simulink model "Practica4"  (R2024b)
settings: Solver=VariableStepAuto  StartTime=0.0  StopTime=1  MaxStep=1e-4  RelTol=1e-3
values from neighbouring files (symbols this model uses):
  C1 = 10e-3    (= 0.01)    [Practica4_Datos.m]    (also in Practica_4.m)
  C2 = 600e-6    (= 0.0006)    [Practica4_Datos.m]    (also in Practica_4.m)
  f = 20e3    (= 20000)    [ApartadoB.m]    (also in ApartadoB_Datos.m; ApartadoC.m = 8000; Practica4_Datos.m = 16000; Practica_4.m = 16000)
  L = 4e-3    (= 0.004)    [ApartadoB.m]    (also in ApartadoB_Datos.m; Practica4_Datos.m = 0.005; Practica_4.m = 0.005)
  L1 = 0    [ApartadoC.m]    (also in Practica4_Datos.m; Practica_4.m)
  L2 = 0    [ApartadoC.m]    (also in Practica4_Datos.m; Practica_4.m)
  Lm = 0    [ApartadoC.m]    (also in Practica4_Datos.m; Practica_4.m)
  Pmp = 10524.2    [ApartadoC.m]    (also in Practica4_Datos.m = 4037.5; Practica_4.m = 4037.5)
  R1 = 0.1    [ApartadoC.m]    (also in Practica4_Datos.m; Practica_4.m)
  R2 = 0.1    [ApartadoC.m]    (also in Practica4_Datos.m; Practica_4.m)
  RL = VdcLinkDes.^2/Pnom    [Practica4_Datos.m]    (also in Practica_4.m)
  Rm = 10e6    (= 10000000)    [ApartadoC.m]    (also in Practica4_Datos.m; Practica_4.m)
  T = 1/f    (= 5e-05)    [ApartadoB.m]    (also in ApartadoB_Datos.m; ApartadoC.m = 0.000125; Practica4_Datos.m = 6.25e-05; Practica_4.m = 6.25e-05)
  V1 = V2/2    (= 200)    [ApartadoC.m]    (also in Practica4_Datos.m; Practica_4.m)
  V2 = 400    [ApartadoC.m]    (also in Practica4_Datos.m; Practica_4.m)
  VdcLinkDes = 800    [Practica4_Datos.m]    (also in Practica_4.m)
  Vmp = 223.836    [ApartadoC.m]    (also in Practica4_Datos.m = 207; Practica_4.m = 207)
libraries: spsParallelRLCBranchLib x9, spsDiodeLib x8, spsCurrentMeasurementLib x6, spsVoltageMeasurementLib x3, slpidlib x2, spsIGBTLib x2, simulink x2, spsLinearTransformerLib x1, spsBistableLib x1, spsPVArrayLib x1, spsThreePhaseProgrammableVoltageSourceLib x1, sps_lib x1
settings Model: Creator=javier  LastModifiedBy=javier

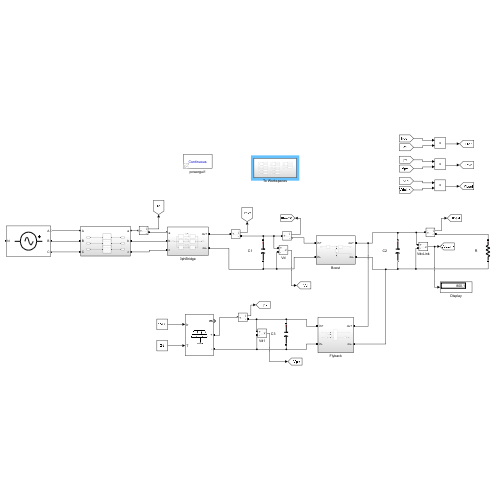
[thumbnail: Simulink's stored preview of the top-level diagram]
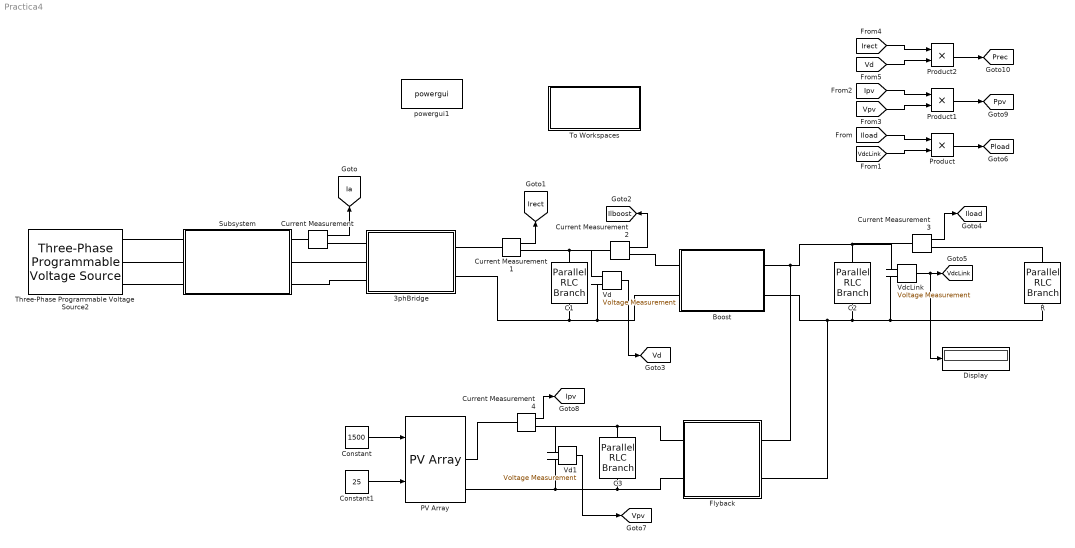
== system Practica4 ==
  3phBridge : Subsystem
  Boost : Subsystem
  C1 : spsParallelRLCBranchLib/Parallel RLC Branch  LConnTagsString=a  RConnTagsString=__new0  BranchType=C  Resistance=30  Inductance=1e-3  SetiL0=off  InitialCurrent=0  Capacitance=C1  Setx0=on  InitialVoltage=VoC1  Measurements=None
  C2 : spsParallelRLCBranchLib/Parallel RLC Branch  LConnTagsString=a  RConnTagsString=__new0  BranchType=C  Resistance=30  Inductance=1e-3  SetiL0=off  InitialCurrent=0  Capacitance=C2  Setx0=on  InitialVoltage=VoC2  Measurements=None
  C3 : spsParallelRLCBranchLib/Parallel RLC Branch  LConnTagsString=a  RConnTagsString=__new0  BranchType=C  Resistance=30  Inductance=1e-3  SetiL0=off  InitialCurrent=0  Capacitance=1.5e-3  Setx0=off  InitialVoltage=0  Measurements=None
  Constant : Constant  Value=1500
  Constant1 : Constant  Value=25
  Current Measurement{,1..4} (5 alike) : spsCurrentMeasurementLib/Current Measurement  PhasorSimulation=off  OutputType=Complex  PSBequivalent=0
  Display : Display
  Flyback : Subsystem
  PV Array : spsPVArrayLib/PV Array  Npar=3  Nser=6  PlotType=array @ 25 deg.C & specified irradiances  S_vec=[1500]  Temp_C_vec=[25]  ModuleName=Advance Solar Hydro Wind Power API-150  PlotWhenSelected=off  Pm=150.075  Ncell=72  Voc=41.8  Isc=5.05  Vm=34.5  Im=4.35  beta_Voc_pc=-0.419  alpha_Isc_pc=0.096  beta_Voc=-0.17514  alpha_Isc=0.004848  IL=5.0762  I0=1.155e-09  nI=1.0233  Rsh=71.9537  Rs=0.37337  RobustModel=off  RobustCellTemperature=313.3991  BAL=on  Tc=1e-6  Tfilter=5e-5
  Product : Product
  Product1 : Product
  Product2 : Product
  R : spsParallelRLCBranchLib/Parallel RLC Branch  LConnTagsString=a  RConnTagsString=__new0  BranchType=R  Resistance=RL  Inductance=1e-3  SetiL0=off  InitialCurrent=0  Capacitance=10e-3  Setx0=off  InitialVoltage=0  Measurements=None
  Subsystem : Subsystem
  Three-Phase Programmable Voltage Source2 : spsThreePhaseProgrammableVoltageSourceLib/Three-Phase Programmable Voltage Source  PositiveSequence="[400  0 50]"  VariationEntity=None  VariationType=Table of time-amplitude pairs  VariationTypeAlt=Step  VariationStep=0.5  VariationRate=10  VariationMagnitude=0.3  VariationFrequency=2  VariationTiming=[1 2]  VariationPhaseA=off  Amplitudes=[1 0.8 1.2 1.0]  TimeValues=[0 0.1 0.15 0.2]  HarmonicGeneration=off  HarmonicA=[3 0.2 -25 0]  HarmonicB=[2 0.15 35 2]  Timing="[0.05  3]"  BusType=swing  Pref=0  Qref=0  Qmin=-inf  Qmax=inf
  To Workspaces : Subsystem
  Vd : spsVoltageMeasurementLib/Voltage Measurement  PhasorSimulation=off  OutputType=Complex  PSBequivalent=0
  Vd1 : spsVoltageMeasurementLib/Voltage Measurement  PhasorSimulation=off  OutputType=Complex  PSBequivalent=0
  VdcLink : spsVoltageMeasurementLib/Voltage Measurement  PhasorSimulation=off  OutputType=Complex  PSBequivalent=0
  powergui1 : sps_lib/powergui  Priority=1  SimulationMode=Continuous  SampleTime=50e-6  frequency=60  Iterations=50  frequencyindice=0  Pbase=100e6  ErrMax=1e-4  UnitsV=kV  UnitsW=MW  buscounter=0  FunctionMessages=off  echomessages=off  EnableUseOfTLC=off  CurrentSourceSwitches=off  DisableSnubberDevices=on  DisableRonSwitches=off  DisableVfSwitches=off  DisplayEquations=off  AutomaticDiscreteSolvers=off  SolverType=Tustin/Backward Euler (TBE)  Interpol=off  ExternalGateDelay=off  methode=off  Ts=100  x0status=blocks  SPID=on  SwTol=0  HookPort=off  NonlinearTolerance=1e-4  nMaxIteration=100  ContinueOnMaxIteration=off  RestoreLinks=warning  ResistiveCurrentMeasurement=off  Frange=[0:2:500]  Ylog=off  Xlog=on  ShowGrid=off  save=off  variable=ZData  structure=0  ZoomFFT=off  StartTime=0.0  cycles=1  DisplayStyle=1  fundamental=60  FreqAxis=off  MaxFrequency=1000  frequencyindicesteady=1  RmsSteady=1  display=off
  tag scope: Ia=global, Ilboost=global, Iload=global, Ipv=global, Irect=global, Pload=global, Ppv=global, Prec=global, Vd=global, VdcLink=global, Vpv=global
  wires:
  Current Measurement/1 -> [Ia]
  Current Measurement1/1 -> [Irect]
  Current Measurement2/1 -> [Ilboost]
  Vd/1 -> [Vd]
  Current Measurement3/1 -> [Iload]
  VdcLink/1 -> Display/1, [VdcLink]
  [Iload] -> Product/1
  [VdcLink] -> Product/2
  Product/1 -> [Pload]
  Constant1/1 -> PV Array/2
  Constant/1 -> PV Array/1
  Vd1/1 -> [Vpv]
  Current Measurement4/1 -> [Ipv]
  Product1/1 -> [Ppv]
  [Vpv] -> Product1/2
  [Ipv] -> Product1/1
  [Irect] -> Product2/1
  [Vd] -> Product2/2
  Product2/1 -> [Prec]
  connections:
  Subsystem/RConn1 -- Three-Phase Programmable Voltage Source2/RConn1
  Subsystem/RConn2 -- Three-Phase Programmable Voltage Source2/RConn2
  Subsystem/RConn3 -- Three-Phase Programmable Voltage Source2/RConn3
  3phBridge/LConn2 -- Subsystem/LConn2
  3phBridge/LConn3 -- Subsystem/LConn3
  Current Measurement/LConn1 -- Subsystem/LConn1
  Current Measurement/RConn1 -- 3phBridge/LConn1
  Current Measurement1/LConn1 -- 3phBridge/RConn1
  C1/LConn1 -- Current Measurement2/LConn1 -- Vd/LConn1 -- Current Measurement1/RConn1
  C1/RConn1 -- Vd/LConn2 -- Boost/LConn2 -- 3phBridge/RConn2
  Current Measurement2/RConn1 -- Boost/LConn1
  Boost/RConn1 -- Flyback/RConn1 -- VdcLink/LConn1 -- Current Measurement3/LConn1 -- C2/LConn1
  R/LConn1 -- Current Measurement3/RConn1
  C2/RConn1 -- R/RConn1 -- VdcLink/LConn2 -- Flyback/RConn2 -- Boost/RConn2
  Flyback/LConn1 -- Vd1/LConn1 -- Current Measurement4/RConn1 -- C3/LConn1
  PV Array/RConn2 -- Vd1/LConn2 -- Flyback/LConn2 -- C3/RConn1
  Current Measurement4/LConn1 -- PV Array/RConn1

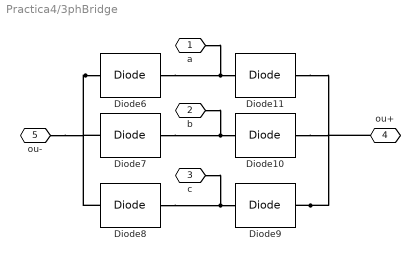
== system Practica4/3phBridge ==
  Diode{6..11} (6 alike) : spsDiodeLib/Diode  Ron=0.001  Lon=0  Vf=0.8  IC=0  UseSnubber=0  Rs=500  Cs=250e-9  Measurements=off
  a : PMIOPort  Side=Left
  b : PMIOPort  Port=2  Side=Left
  c : PMIOPort  Port=3  Side=Left
  ou+ : PMIOPort  Port=4  Side=Right
  ou- : PMIOPort  Port=5  Side=Right
  connections:
  Diode7/RConn1 -- b/RConn1 -- Diode10/LConn1
  Diode9/RConn1 -- ou+/RConn1 -- Diode10/RConn1 -- Diode11/RConn1
  Diode6/RConn1 -- a/RConn1 -- Diode11/LConn1
  Diode8/RConn1 -- c/RConn1 -- Diode9/LConn1
  Diode6/LConn1 -- ou-/RConn1 -- Diode8/LConn1 -- Diode7/LConn1

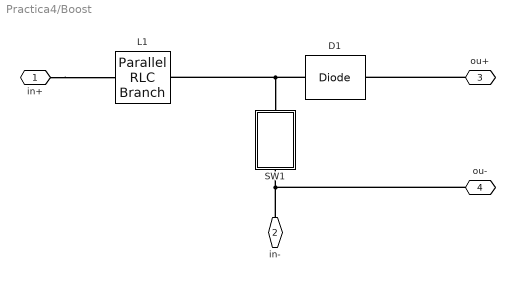
== system Practica4/Boost ==
  D1 : spsDiodeLib/Diode  Ron=0.001  Lon=0  Vf=0.8  IC=0  UseSnubber=0  Rs=500  Cs=250e-9  Measurements=off
  L1 : spsParallelRLCBranchLib/Parallel RLC Branch  LConnTagsString=a  RConnTagsString=__new0  BranchType=L  Resistance=1  Inductance=8e-3  SetiL0=off  InitialCurrent=0  Capacitance=1e-6  Setx0=off  InitialVoltage=0  Measurements=None
  SW1 : Subsystem
  in+ : PMIOPort  Side=Left
  in- : PMIOPort  Port=2  Side=Left
  ou+ : PMIOPort  Port=3  Side=Right
  ou- : PMIOPort  Port=4  Side=Right
  connections:
  D1/LConn1 -- SW1/LConn1 -- L1/RConn1
  ou+/RConn1 -- D1/RConn1
  in-/RConn1 -- SW1/RConn1 -- ou-/RConn1
  in+/RConn1 -- L1/LConn1

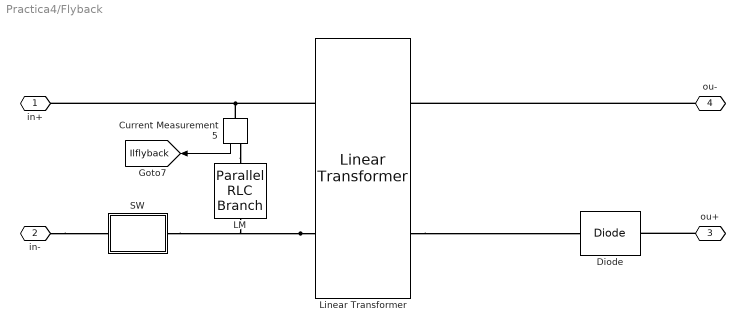
== system Practica4/Flyback ==
  Current Measurement5 : spsCurrentMeasurementLib/Current Measurement  PhasorSimulation=off  OutputType=Complex  PSBequivalent=0
  Diode : spsDiodeLib/Diode  Ron=0.001  Lon=0  Vf=0.8  IC=0  UseSnubber=0  Rs=500  Cs=250e-9  Measurements=off
  LM : spsParallelRLCBranchLib/Parallel RLC Branch  LConnTagsString=a  RConnTagsString=__new0  BranchType=L  Resistance=1  Inductance=6e-3  SetiL0=off  InitialCurrent=0  Capacitance=1.5e-3  Setx0=off  InitialVoltage=0  Measurements=None
  Linear Transformer : spsLinearTransformerLib/Linear Transformer  UNITS=SI  NominalPower=[Pmp f ]  winding1=[V1 R1 L1]  winding2=[V2 R2 L2]  ThreeWindings=off  winding3=[3.15e+05 0.7938 0.084225]  RmLm=[Rm Lm]  Measurements=None  DataType=on
  SW : Subsystem
  in+ : PMIOPort  Side=Left
  in- : PMIOPort  Port=2  Side=Left
  ou+ : PMIOPort  Port=3  Side=Right
  ou- : PMIOPort  Port=4  Side=Right
  tag scope: Ilflyback=global
  wires:
  Current Measurement5/1 -> [Ilflyback]
  connections:
  in-/RConn1 -- SW/RConn1
  Linear Transformer/RConn2 -- Diode/LConn1
  ou+/RConn1 -- Diode/RConn1
  Current Measurement5/LConn1 -- in+/RConn1 -- Linear Transformer/LConn1
  Linear Transformer/LConn2 -- SW/LConn1 -- LM/RConn1
  Current Measurement5/RConn1 -- LM/LConn1
  ou-/RConn1 -- Linear Transformer/RConn1

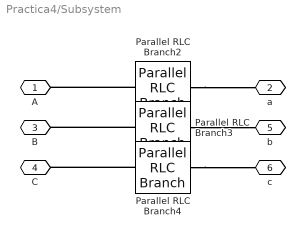
== system Practica4/Subsystem ==
  Parallel RLC Branch2 : spsParallelRLCBranchLib/Parallel RLC Branch  LConnTagsString=a  RConnTagsString=__new0  BranchType=L  Resistance=30  Inductance=5e-3  SetiL0=off  InitialCurrent=0  Capacitance=1e-6  Setx0=off  InitialVoltage=0  Measurements=None
  Parallel RLC Branch3 : spsParallelRLCBranchLib/Parallel RLC Branch  LConnTagsString=a  RConnTagsString=__new0  BranchType=L  Resistance=30  Inductance=L  SetiL0=off  InitialCurrent=0  Capacitance=1e-6  Setx0=off  InitialVoltage=0  Measurements=None
  Parallel RLC Branch4 : spsParallelRLCBranchLib/Parallel RLC Branch  LConnTagsString=a  RConnTagsString=__new0  BranchType=L  Resistance=30  Inductance=L  SetiL0=off  InitialCurrent=0  Capacitance=1e-6  Setx0=off  InitialVoltage=0  Measurements=None
  A : PMIOPort  Side=Right
  a : PMIOPort  Port=2  Side=Left
  B : PMIOPort  Port=3  Side=Right
  C : PMIOPort  Port=4  Side=Right
  b : PMIOPort  Port=5  Side=Left
  c : PMIOPort  Port=6  Side=Left
  connections:
  Parallel RLC Branch2/RConn1 -- A/RConn1
  Parallel RLC Branch4/RConn1 -- C/RConn1
  Parallel RLC Branch2/LConn1 -- a/RConn1
  Parallel RLC Branch4/LConn1 -- c/RConn1
  Parallel RLC Branch3/LConn1 -- b/RConn1
  Parallel RLC Branch3/RConn1 -- B/RConn1

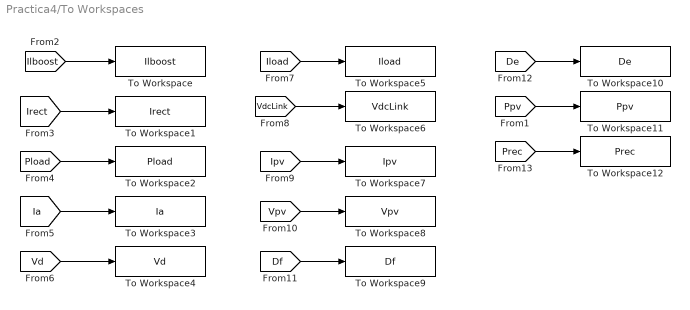
== system Practica4/To Workspaces ==
  To Workspace : ToWorkspace  VariableName=Ilboost  SaveFormat=Timeseries  SampleTime=-1
  To Workspace1 : ToWorkspace  VariableName=Irect  SaveFormat=Timeseries  SampleTime=-1
  To Workspace10 : ToWorkspace  VariableName=De  SaveFormat=Timeseries  SampleTime=-1
  To Workspace11 : ToWorkspace  VariableName=Ppv  SaveFormat=Timeseries  SampleTime=-1
  To Workspace12 : ToWorkspace  VariableName=Prec  SaveFormat=Timeseries  SampleTime=-1
  To Workspace2 : ToWorkspace  VariableName=Pload  SaveFormat=Timeseries  SampleTime=-1
  To Workspace3 : ToWorkspace  VariableName=Ia  SaveFormat=Timeseries  SampleTime=-1
  To Workspace4 : ToWorkspace  VariableName=Vd  SaveFormat=Timeseries  SampleTime=-1
  To Workspace5 : ToWorkspace  VariableName=Iload  SaveFormat=Timeseries  SampleTime=-1
  To Workspace6 : ToWorkspace  VariableName=VdcLink  SaveFormat=Timeseries  SampleTime=-1
  To Workspace7 : ToWorkspace  VariableName=Ipv  SaveFormat=Timeseries  SampleTime=-1
  To Workspace8 : ToWorkspace  VariableName=Vpv  SaveFormat=Timeseries  SampleTime=-1
  To Workspace9 : ToWorkspace  VariableName=Df  SaveFormat=Timeseries  SampleTime=-1
  wires:
  [Ia] -> To Workspace3/1
  [Vd] -> To Workspace4/1
  [Iload] -> To Workspace5/1
  [Ipv] -> To Workspace7/1
  [Ilboost] -> To Workspace/1
  [Df] -> To Workspace9/1
  [De] -> To Workspace10/1
  [VdcLink] -> To Workspace6/1
  [Pload] -> To Workspace2/1
  [Irect] -> To Workspace1/1
  [Vpv] -> To Workspace8/1
  [Ppv] -> To Workspace11/1
  [Prec] -> To Workspace12/1

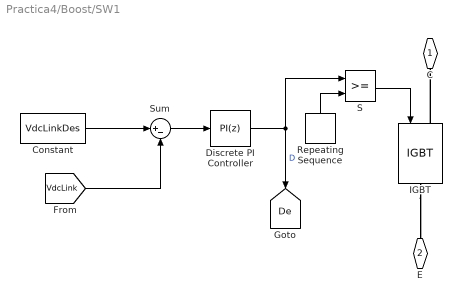
== system Practica4/Boost/SW1 ==
  Constant : Constant  Value=VdcLinkDes
  Discrete PI Controller : slpidlib/PID Controller  Controller=PI  Form=Ideal  TimeDomain=Discrete-time  UseExternalTs=off  SampleTime=T/2  IntegratorMethod=Forward Euler  FilterMethod=Forward Euler  ControllerParametersSource=internal  P=0.0001  I=80  UseKiTs=off  D=0  UseExternalDerivativeSource=off  N=100  UseFilter=on  TunerSelectOption=Transfer Function Based (PID Tuner App)  InitialConditionSource=internal  InitialConditionForIntegrator=0  InitialConditionForFilter=0  DifferentiatorICPrevScaledInput=0  ExternalReset=none  TrackingMode=off  Kt=1  LimitOutput=off  SatLimitsSource=internal  UpperSaturationLimit=inf  LowerSaturationLimit=-inf  LinearizeAsGain=off  AntiWindupMode=none  Kb=1  LimitIntegrator=off  UpperIntegratorSaturationLimit=inf  LowerIntegratorSaturationLimit=-inf  POutMin=[]  POutMax=[]  IOutMin=[]  IOutMax=[]  DOutMin=[]  DOutMax=[]  NOutMin=[]  NOutMax=[]  SumOutMin=[]  SumOutMax=[]  SaturationOutMin=[]  SaturationOutMax=[]  PParamMin=[]  PParamMax=[]  IParamMin=[]  IParamMax=[]  DParamMin=[]  DParamMax=[]  NParamMin=[]  NParamMax=[]  KbParamMin=[]  KbParamMax=[]  KtParamMin=[]  KtParamMax=[]  KbOutMin=[]  KbOutMax=[]  KtOutMin=[]  KtOutMax=[]  IntegratorOutMin=[]  IntegratorOutMax=[]  FilterOutMin=[]  FilterOutMax=[]  SumI1OutMin=[]  SumI1OutMax=[]  SumI2OutMin=[]  SumI2OutMax=[]  SumI3OutMin=[]  SumI3OutMax=[]  SumI4OutMin=[]  SumI4OutMax=[]  SumDOutMin=[]  SumDOutMax=[]  DifferentiatorOutMin=[]  DifferentiatorOutMax=[]  FilterDiffOutCoefMin=[]  FilterDiffOutCoefMax=[]  ReciprocalOutMin=[]  ReciprocalOutMax=[]  SumDenOutMin=[]  SumDenOutMax=[]  SumNumOutMin=[]  SumNumOutMax=[]  DivideOutMin=[]  DivideOutMax=[]  UdiffTsProdOutMin=[]  UdiffTsProdOutMax=[]  NTsProdOutMin=[]  NTsProdOutMax=[]  UintegralTsProdOutMin=[]  UintegralTsProdOutMax=[]  UngainTsProdOutMin=[]  UngainTsProdOutMax=[]  ClampingZeroOutDataTypeStr=Inherit: Inherit via back propagation  ClampingZeroOutMin=[]  ClampingZeroOutMax=[]  FilterDenConstantOutDataTypeStr=Inherit: Inherit via back propagation  FilterDenConstantOutMin=[]  FilterDenConstantOutMax=[]  PCopyOutDataTypeStr=Inherit: Inherit via back propagation  PCopyOutMin=[]  PCopyOutMax=[]  NCopyOutDataTypeStr=Inherit: Inherit via back propagation  NCopyOutMin=[]  NCopyOutMax=[]  IntegratorContinuousStateAttributes=''  IntegratorStateMustResolveToSignalObject=off  IntegratorRTWStateStorageClass=Auto  FilterContinuousStateAttributes=''  FilterStateMustResolveToSignalObject=off  FilterRTWStateStorageClass=Auto  ParallelPVariant=Passthrough  IdealPVariant=InternalParameters  IVariant=InternalParameters  DVariant=Disabled  IntegratorVariant=Discrete  SatVariant=Disabled  AWVariant=Passthrough  PCopyVariant=Disabled  TRVariant=Disabled  FdbkBlocksVariant=Forward  IdealPFdbkVariant=Disabled  SatFdbkVariant=Disabled  DerivativeFilterVariant=Disabled  NVariant=Disabled  NCopyVariant=Disabled_SignalSpec  FilterICVariant=Disabled  IntegratorICVariant=InternalICs  ExternalResetVariant=Disabled  TRSumVariant=Passthrough  SumFdbkVariant=Disabled  SumVariant=Sum_PI  TsampFilterVariant=InternalTs  TsampNgainVariant=Passthrough  TsampIntegralVariant=Disabled_SignalSpec  ExternalSaturationOutDataTypeStr=Inherit: Same as second input  DerivativeSourceVariant=Disabled  PreIntVariant=InternalPreInt
      settings: LibrarySourceBlock=simulink/Discrete/Discrete PID Controller
  IGBT : spsIGBTLib/IGBT  Ron=0.001  Lon=0  Vf=1  Tf=1e-6  Tt=2e-6  IC=0  Rs=1e5  Cs=inf  Measurements=off
  Repeating Sequence : simulink/Sources/Repeating Sequence  rep_seq_t=RepeatingTime  rep_seq_y=RepeatingOut
  S : RelationalOperator  OutDataTypeStr=boolean  RndMeth=Simplest  InputSameDT=off
  Sum : Sum  Inputs=|+-
  C : PMIOPort  Side=Left
  E : PMIOPort  Port=2  Side=Right
  tag scope: De=global
  wires:
  S/1 -> IGBT/1
  Discrete PI Controller/1 -> [De], S/1  "D"
  Repeating Sequence/1 -> S/2
  Sum/1 -> Discrete PI Controller/1
  Constant/1 -> Sum/1
  [VdcLink] -> Sum/2
  connections:
  IGBT/RConn1 -- E/RConn1
  IGBT/LConn1 -- C/RConn1

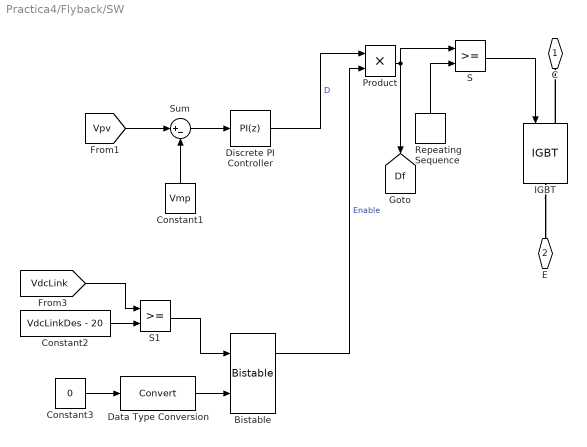
== system Practica4/Flyback/SW ==
  Bistable : spsBistableLib/Bistable  Qpriority=Set  ic=0  Ts=0
  Constant1 : Constant  Value=Vmp
  Constant2 : Constant  Value=VdcLinkDes - 20
  Constant3 : Constant  Value=0
  Data Type Conversion : DataTypeConversion  SaturateOnIntegerOverflow=off  RndMeth=Floor
  Discrete PI Controller : slpidlib/PID Controller  Controller=PI  Form=Ideal  TimeDomain=Discrete-time  UseExternalTs=off  SampleTime=T/2  IntegratorMethod=Forward Euler  FilterMethod=Forward Euler  ControllerParametersSource=internal  P=0.005  I=50  UseKiTs=off  D=0  UseExternalDerivativeSource=off  N=100  UseFilter=on  TunerSelectOption=Transfer Function Based (PID Tuner App)  InitialConditionSource=internal  InitialConditionForIntegrator=0  InitialConditionForFilter=0  DifferentiatorICPrevScaledInput=0  ExternalReset=none  TrackingMode=off  Kt=1  LimitOutput=off  SatLimitsSource=internal  UpperSaturationLimit=inf  LowerSaturationLimit=-inf  LinearizeAsGain=off  AntiWindupMode=none  Kb=1  LimitIntegrator=off  UpperIntegratorSaturationLimit=inf  LowerIntegratorSaturationLimit=-inf  POutMin=[]  POutMax=[]  IOutMin=[]  IOutMax=[]  DOutMin=[]  DOutMax=[]  NOutMin=[]  NOutMax=[]  SumOutMin=[]  SumOutMax=[]  SaturationOutMin=[]  SaturationOutMax=[]  PParamMin=[]  PParamMax=[]  IParamMin=[]  IParamMax=[]  DParamMin=[]  DParamMax=[]  NParamMin=[]  NParamMax=[]  KbParamMin=[]  KbParamMax=[]  KtParamMin=[]  KtParamMax=[]  KbOutMin=[]  KbOutMax=[]  KtOutMin=[]  KtOutMax=[]  IntegratorOutMin=[]  IntegratorOutMax=[]  FilterOutMin=[]  FilterOutMax=[]  SumI1OutMin=[]  SumI1OutMax=[]  SumI2OutMin=[]  SumI2OutMax=[]  SumI3OutMin=[]  SumI3OutMax=[]  SumI4OutMin=[]  SumI4OutMax=[]  SumDOutMin=[]  SumDOutMax=[]  DifferentiatorOutMin=[]  DifferentiatorOutMax=[]  FilterDiffOutCoefMin=[]  FilterDiffOutCoefMax=[]  ReciprocalOutMin=[]  ReciprocalOutMax=[]  SumDenOutMin=[]  SumDenOutMax=[]  SumNumOutMin=[]  SumNumOutMax=[]  DivideOutMin=[]  DivideOutMax=[]  UdiffTsProdOutMin=[]  UdiffTsProdOutMax=[]  NTsProdOutMin=[]  NTsProdOutMax=[]  UintegralTsProdOutMin=[]  UintegralTsProdOutMax=[]  UngainTsProdOutMin=[]  UngainTsProdOutMax=[]  ClampingZeroOutDataTypeStr=Inherit: Inherit via back propagation  ClampingZeroOutMin=[]  ClampingZeroOutMax=[]  FilterDenConstantOutDataTypeStr=Inherit: Inherit via back propagation  FilterDenConstantOutMin=[]  FilterDenConstantOutMax=[]  PCopyOutDataTypeStr=Inherit: Inherit via back propagation  PCopyOutMin=[]  PCopyOutMax=[]  NCopyOutDataTypeStr=Inherit: Inherit via back propagation  NCopyOutMin=[]  NCopyOutMax=[]  IntegratorContinuousStateAttributes=''  IntegratorStateMustResolveToSignalObject=off  IntegratorRTWStateStorageClass=Auto  FilterContinuousStateAttributes=''  FilterStateMustResolveToSignalObject=off  FilterRTWStateStorageClass=Auto  ParallelPVariant=Passthrough  IdealPVariant=InternalParameters  IVariant=InternalParameters  DVariant=Disabled  IntegratorVariant=Discrete  SatVariant=Disabled  AWVariant=Passthrough  PCopyVariant=Disabled  TRVariant=Disabled  FdbkBlocksVariant=Forward  IdealPFdbkVariant=Disabled  SatFdbkVariant=Disabled  DerivativeFilterVariant=Disabled  NVariant=Disabled  NCopyVariant=Disabled_SignalSpec  FilterICVariant=Disabled  IntegratorICVariant=InternalICs  ExternalResetVariant=Disabled  TRSumVariant=Passthrough  SumFdbkVariant=Disabled  SumVariant=Sum_PI  TsampFilterVariant=InternalTs  TsampNgainVariant=Passthrough  TsampIntegralVariant=Disabled_SignalSpec  ExternalSaturationOutDataTypeStr=Inherit: Same as second input  DerivativeSourceVariant=Disabled  PreIntVariant=InternalPreInt
  IGBT : spsIGBTLib/IGBT  Ron=0.001  Lon=0  Vf=1  Tf=1e-6  Tt=2e-6  IC=0  Rs=1e5  Cs=inf  Measurements=off
  Product : Product
  Repeating Sequence : simulink/Sources/Repeating Sequence  rep_seq_t=RepeatingTime  rep_seq_y=RepeatingOut
  S : RelationalOperator  OutDataTypeStr=boolean  RndMeth=Simplest  InputSameDT=off
  S1 : RelationalOperator  OutDataTypeStr=boolean  RndMeth=Simplest  InputSameDT=off
  Sum : Sum  Inputs=|+-
  C : PMIOPort  Side=Left
  E : PMIOPort  Port=2  Side=Right
  tag scope: Df=global
  wires:
  Discrete PI Controller/1 -> Product/1  "D"
  Sum/1 -> Discrete PI Controller/1
  [Vpv] -> Sum/1
  Constant1/1 -> Sum/2
  Constant3/1 -> Data Type Conversion/1
  [VdcLink] -> S1/1
  Data Type Conversion/1 -> Bistable/2
  S1/1 -> Bistable/1
  Constant2/1 -> S1/2
  Bistable/1 -> Product/2  "Enable"
  Product/1 -> S/1, [Df]
  Repeating Sequence/1 -> S/2
  S/1 -> IGBT/1
  connections:
  IGBT/RConn1 -- E/RConn1
  IGBT/LConn1 -- C/RConn1
